simulink model "dual_motor_pitch_mpc"  (R2021b)
settings: Solver=ode45  StartTime=0.0  StopTime=100  MaxStep=1e-3  RelTol=1e-6  AbsTol=1e-8
settings Model: Creator=xuan1  LastModifiedBy=xuan1

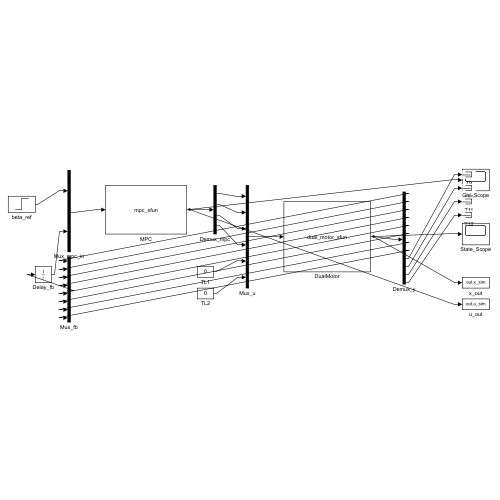
[thumbnail: Simulink's stored preview of the top-level diagram]
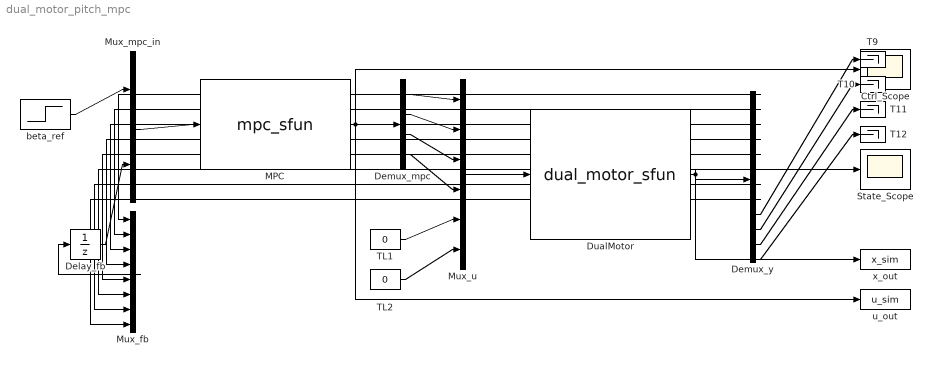
== system dual_motor_pitch_mpc ==
  Ctrl_Scope : Scope
  Delay_fb : UnitDelay  SampleTime=0.01  HasFrameUpgradeWarning=on
  Demux_mpc : Demux
  Demux_y : Demux  Outputs=12
  DualMotor : S-Function  FunctionName=dual_motor_sfun  SFunctionDeploymentMode=off  EnableBusSupport=off
  MPC : S-Function  FunctionName=mpc_sfun  SFunctionDeploymentMode=off  EnableBusSupport=off
  Mux_fb : Mux  Inputs=8
  Mux_mpc_in : Mux  Inputs=[1, 8]
  Mux_u : Mux  Inputs=6
  State_Scope : Scope
  T{9..12} (4 alike) : Terminator
  TL1 : Constant  Value=0
  TL2 : Constant  Value=0
  beta_ref : Step  Time=30  After=15  SampleTime=0
  u_out : ToWorkspace  VariableName=u_sim  SaveFormat=Timeseries  SampleTime=-1
  x_out : ToWorkspace  VariableName=x_sim  SaveFormat=Timeseries  SampleTime=-1
  wires:
  beta_ref/1 -> Mux_mpc_in/1
  Mux_mpc_in/1 -> MPC/1
  MPC/1 -> Demux_mpc/1, Ctrl_Scope/1, u_out/1
  Demux_mpc/1 -> Mux_u/1
  Demux_mpc/2 -> Mux_u/2
  Demux_mpc/3 -> Mux_u/3
  Demux_mpc/4 -> Mux_u/4
  TL1/1 -> Mux_u/5
  TL2/1 -> Mux_u/6
  Mux_u/1 -> DualMotor/1
  DualMotor/1 -> Demux_y/1, State_Scope/1, x_out/1
  Demux_y/1 -> Mux_fb/1
  Demux_y/2 -> Mux_fb/2
  Demux_y/3 -> Mux_fb/3
  Demux_y/4 -> Mux_fb/4
  Demux_y/5 -> Mux_fb/5
  Demux_y/6 -> Mux_fb/6
  Demux_y/7 -> Mux_fb/7
  Demux_y/8 -> Mux_fb/8
  Mux_fb/1 -> Delay_fb/1
  Delay_fb/1 -> Mux_mpc_in/2
  Demux_y/9 -> T9/1
  Demux_y/10 -> T10/1
  Demux_y/11 -> T11/1
  Demux_y/12 -> T12/1
